simulink model "Squelette_DSPB_ModulateurOQPSK"  (R2016a)
settings: Solver=FixedStepDiscrete  StartTime=0.0  StopTime=1e-3  RelTol=1e-3
InitFcn:
  | %% DSPBuilder Start
  | alt_dspbuilder_update_model(bdroot)
  | %% DSPBuilder End
libraries: allblocks_alteradspbuilder2 x243
(part 1 of 2)
settings Model: Creator=rhev2401  LastModifiedBy=cous2509
settings DataIOCC: LimitDataPoints=on  SaveFormat=Array  SignalLoggingSaveFormat=ModelDataLogs
settings DebuggingCC: SolverPrmCheckMsg=warning  MultiTaskDSMMsg=warning  MultiTaskCondExecSysMsg=none
settings HardwareCC: ProdBitPerPointer=32  ProdLargestAtomicFloat=None  ProdIntDivRoundTo=Undefined  ProdEndianess=Unspecified  ProdWordSize=32  ProdHWDeviceType=32-bit Generic
settings ModelReferenceCC: PropagateSignalLabelsOutOfModel=off
settings ConfigComp: CovModelRefEnable=Off  CovSFcnEnable=off

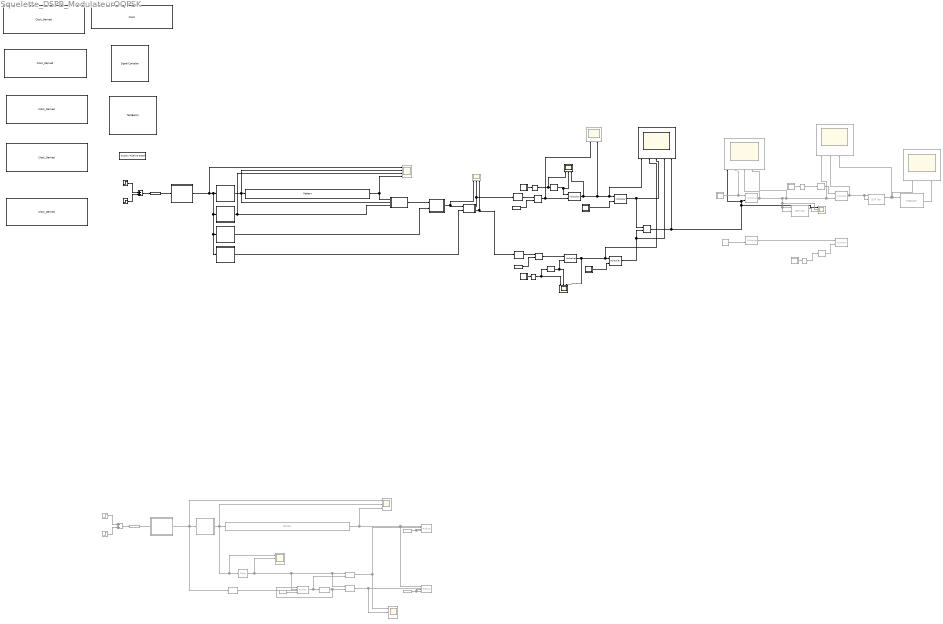
== system Squelette_DSPB_ModulateurOQPSK ==
  note: Transformation de la trame
  note: Rail Q O-QPSK
  note: Rail I O-QPSK
  note: Simulates an event to begin a transmission
  note: Bouton 01
  note: On se crée une impulsion qui dure la longueur de la trame.
      |
      | En vrai, il faudrait transmettre jusqu'à ce que le buffer soit vide...
  note: Paquet à transmettre (chips)
  note: Chipclock
  note: Notez que, pour ce programme, on a choisi d'utiliser la fréquence d'horloge de 100MHz.
  note: Si le dernier chip est rentré sur I, le prochain rentre sur Q, et vice-versa; génération de deux horloges d'1 MHz déphasées
  note: Cette boîte à délai compense pour le délai de la boîte "Pattern" (notez que la sortie de la boîte pattern commence 1 coup de clock après l'apparition du Enable)
  note: Si le dernier chip est rentré sur I, le prochain rentre sur Q, et vice-versa; génération de deux horloges d'1 MHz déphasées
  note: Simulates an event to begin a transmission
  note: 0000000000000000000000000000000011100101 10010000111011111111001101110100000101101110010100110001010100001010000110000110
      | 0 0 0 0 0 0 0 0 7 A 9 0 7 F F C E 2 8 6 7 A C 8 A 0 5 8 1 6
  note: Bouton 01
  note: On se crée une impulsion qui dure la longueur de la trame.
      |
      | En vrai, il faudrait transmettre jusqu'à ce que le buffer soit vide...
  note: Paquet à transmettre
  note: Bitclock
  note: Notez que, pour ce programme, on a choisi d'utiliser la fréquence d'horloge de 100MHz.
  note: Bit to symbol
  note: Symbol to chip
  note: Chip to I/Q
  1MHz Pulse Generator2 : Subsystem
  250kHz Pulse Generator : Subsystem
  2MHz Pulse Generator : Subsystem  Commented=on
  2MHz Pulse Generator2 : Subsystem
  62.5kHz Pulse Generator1 : Subsystem
  Add : Sum  Commented=on
  Add1 : Sum
  Bit to symbol : Subsystem
  Bouton : Subsystem  Commented=on
  Bouton1 : Subsystem
  Chip to I/Q : Subsystem
  Clock_100MHz : allblocks_alteradspbuilder2/Clock_Derived  ClockNumerator=1  ClockDenominator=2  ResetLatency=0  ResetRegisterCascadeDepth=0  SimulationStartCycle=5  PhaseOffset=0  Reset=aclr_100MHz  ResetType=Active Low  Export=off
  Clock_125MHz : allblocks_alteradspbuilder2/Clock_Derived  ClockNumerator=10  ClockDenominator=25  ResetLatency=0  ResetRegisterCascadeDepth=0  SimulationStartCycle=5  PhaseOffset=0  Reset=aclr_125MHz  ResetType=Active Low  Export=off
  Clock_1MHz : allblocks_alteradspbuilder2/Clock_Derived  ClockNumerator=50  ClockDenominator=1  ResetLatency=0  ResetRegisterCascadeDepth=0  SimulationStartCycle=5  PhaseOffset=0  Reset=aclr_1MHz  ResetType=Active Low  Export=off
  Clock_2MHz : allblocks_alteradspbuilder2/Clock_Derived  ClockNumerator=25  ClockDenominator=1  ResetLatency=0  ResetRegisterCascadeDepth=0  SimulationStartCycle=5  PhaseOffset=0  Reset=aclr_2MHz  ResetType=Active Low  Export=off
  Clock_50MHz : allblocks_alteradspbuilder2/Clock  ClockPeriod=20  ClockPeriodUnit=ns  SampleTime=20e-9  ResetLatency=0  ResetRegisterCascadeDepth=0  SimulationStartCycle=5  PhaseOffset=0  Reset=aclr  ResetType=Active Low  Export=off
  Clock_62p5MHz : allblocks_alteradspbuilder2/Clock_Derived  ClockNumerator=800  ClockDenominator=1  ResetLatency=0  ResetRegisterCascadeDepth=0  SimulationStartCycle=5  PhaseOffset=0  Reset=aclr_62p5MHz  ResetType=Active Low  Export=off
  Constant : allblocks_alteradspbuilder2/Constant  Commented=on  mask_cst=1  BusType=Signed Integer  bwl=8  bwr=0  roundMode=Truncate  satMode=Wrap  SpecifyClock=off  allowFloatingPointOverride=on  logOutputs=off  logFile=U:\S6\Projet\Squelette_ModulateurOQPSK__ORIG\tb_Squelette_DSPB_ModulateurOQPSK\Squelette%5FDSPB%5FModulateurOQPSK_Constant.fixedpointlog
  Constant1 : allblocks_alteradspbuilder2/Constant  Commented=on  mask_cst=1  BusType=Signed Integer  bwl=8  bwr=0  roundMode=Truncate  satMode=Wrap  SpecifyClock=off  allowFloatingPointOverride=on  logOutputs=off  logFile=U:\S6\Projet\Squelette_ModulateurOQPSK__ORIG\tb_Squelette_DSPB_ModulateurOQPSK\Squelette%5FDSPB%5FModulateurOQPSK_Constant1.fixedpointlog
  Constant2 : allblocks_alteradspbuilder2/Constant  Commented=on  mask_cst=1  BusType=Signed Integer  bwl=8  bwr=0  roundMode=Truncate  satMode=Wrap  SpecifyClock=off  allowFloatingPointOverride=on  logOutputs=off  logFile=U:\S6\Projet\Squelette_ModulateurOQPSK__ORIG\tb_Squelette_DSPB_ModulateurOQPSK\Squelette%5FDSPB%5FModulateurOQPSK_Constant2.fixedpointlog
  Constant3 : allblocks_alteradspbuilder2/Constant  mask_cst=-1  BusType=Signed Integer  bwl=8  bwr=4  roundMode=Truncate  satMode=Wrap  SpecifyClock=on  clock=Clock_100MHz  allowFloatingPointOverride=on  logOutputs=off  logFile=U:\S6\Projet\Squelette_ModulateurOQPSK__ORIG\tb_Squelette_DSPB_ModulateurOQPSK\Squelette%5FDSPB%5FModulateurOQPSK_Constant3.fixedpointlog
  Constant5 : allblocks_alteradspbuilder2/Constant  mask_cst=-1  BusType=Signed Integer  bwl=8  bwr=4  roundMode=Truncate  satMode=Wrap  SpecifyClock=on  clock=Clock_100MHz  allowFloatingPointOverride=on  logOutputs=off  logFile=U:\S6\Projet\Squelette_ModulateurOQPSK__ORIG\tb_Squelette_DSPB_ModulateurOQPSK\Squelette%5FDSPB%5FModulateurOQPSK_Constant5.fixedpointlog
  Coswave : Subsystem
  Coswave1 : Subsystem  Commented=on
  Delay : allblocks_alteradspbuilder2/Delay  Commented=on  pipeline=1  pipeline_display=1  ClockPhase=1  use_ena=off  use_sclr=off  allowFloatingPointOverride=on  logOutputs=off  logFile=U:\S6\Projet\Squelette_ModulateurOQPSK__ORIG\tb_Squelette_DSPB_ModulateurOQPSK\Squelette%5FDSPB%5FModulateurOQPSK_Delay.fixedpointlog  use_init=off  reset_value=1
  Delay1 : allblocks_alteradspbuilder2/Delay  pipeline=5  pipeline_display=5  ClockPhase=1  use_ena=off  use_sclr=off  allowFloatingPointOverride=on  logOutputs=off  logFile=U:\S6\Projet\Squelette_ModulateurOQPSK__ORIG\tb_Squelette_DSPB_ModulateurOQPSK\Squelette%5FDSPB%5FModulateurOQPSK_Delay1.fixedpointlog  use_init=off  reset_value=1
  Delay2 : allblocks_alteradspbuilder2/Delay  Commented=on  pipeline=5  pipeline_display=5  ClockPhase=1  use_ena=off  use_sclr=off  allowFloatingPointOverride=on  logOutputs=off  logFile=U:\S6\Projet\Squelette_ModulateurOQPSK__ORIG\tb_Squelette_DSPB_ModulateurOQPSK\Squelette%5FDSPB%5FModulateurOQPSK_Delay2.fixedpointlog  use_init=off  reset_value=1
  Delay3 : allblocks_alteradspbuilder2/Delay  Commented=on  pipeline=55  pipeline_display=55  ClockPhase=1  use_ena=off  use_sclr=off  allowFloatingPointOverride=on  logOutputs=off  logFile=U:\S6\Projet\Squelette_ModulateurOQPSK__ORIG\tb_Squelette_DSPB_ModulateurOQPSK\Squelette%5FDSPB%5FModulateurOQPSK_Delay3.fixedpointlog  use_init=off  reset_value=1
  Delay4 : allblocks_alteradspbuilder2/Delay  pipeline=55  pipeline_display=55  ClockPhase=1  use_ena=off  use_sclr=off  allowFloatingPointOverride=on  logOutputs=off  logFile=U:\S6\Projet\Squelette_ModulateurOQPSK__ORIG\tb_Squelette_DSPB_ModulateurOQPSK\Squelette%5FDSPB%5FModulateurOQPSK_Delay4.fixedpointlog  use_init=off  reset_value=1
  Display Pipeline Depth : allblocks_alteradspbuilder2/Display Pipeline Depth  DisplayLatencyOnBlocks=on
  Flipflop : allblocks_alteradspbuilder2/Flipflop  Commented=on  mode=DFFE  BusType=Single Bit  bwl=2  bwr=2  pipeline_display=1
  Flipflop1 : allblocks_alteradspbuilder2/Flipflop  Commented=on  mode=DFFE  BusType=Single Bit  bwl=2  bwr=2  pipeline_display=1
  Flipflop2 : allblocks_alteradspbuilder2/Flipflop  Commented=on  mode=DFFE  BusType=Single Bit  bwl=2  bwr=2  pipeline_display=1
  Gain : allblocks_alteradspbuilder2/Gain  vgain=2  BusType=Signed Integer  bwl=6  bwr=0  pipeline=0  pipeline_display=0  allowFloatingPointOverride=on  logOutputs=off  logFile=U:\S6\Projet\Squelette_ModulateurOQPSK__ORIG\tb_Squelette_DSPB_ModulateurOQPSK\Squelette%5FDSPB%5FModulateurOQPSK_Gain.fixedpointlog  use_ena=off  use_aclr=off  lpm=off  MaskValue=1
  Gain1 : allblocks_alteradspbuilder2/Gain  vgain=2  BusType=Signed Integer  bwl=6  bwr=0  pipeline=0  pipeline_display=0  allowFloatingPointOverride=on  logOutputs=off  logFile=U:\S6\Projet\Squelette_ModulateurOQPSK__ORIG\tb_Squelette_DSPB_ModulateurOQPSK\Squelette%5FDSPB%5FModulateurOQPSK_Gain1.fixedpointlog  use_ena=off  use_aclr=off  lpm=off  MaskValue=1
  Input : allblocks_alteradspbuilder2/Input  Commented=on  iofile=U:\S6\Projet\Squelette_ModulateurOQPSK__ORIG\tb_Squelette_DSPB_ModulateurOQPSK\Squelette%5FDSPB%5FModulateurOQPSK_Input.salt  BusType=Single Bit  bwl=1  bwr=0  SpecifyClock=on  clock=Clock_100MHz  PORTTYPE=Input  externalType=Inferred  allowFloatingPointOverride=on  logOutputs=off
  Input1 : allblocks_alteradspbuilder2/Input  iofile=U:\S6\Projet\Squelette_ModulateurOQPSK__ORIG\tb_Squelette_DSPB_ModulateurOQPSK\Squelette%5FDSPB%5FModulateurOQPSK_Input1.salt  BusType=Single Bit  bwl=1  bwr=0  SpecifyClock=on  clock=Clock_100MHz  PORTTYPE=Input  externalType=Inferred  allowFloatingPointOverride=on  logOutputs=off
  Integrator : allblocks_alteradspbuilder2/Integrator  Commented=on  bwl=32  depth=32  pipeline_display=32  use_ena=off  use_sclr=on  allowFloatingPointOverride=on  logOutputs=off  logFile=U:\S6\Projet\Squelette_ModulateurOQPSK__ORIG\tb_Squelette_DSPB_ModulateurOQPSK\Squelette%5FDSPB%5FModulateurOQPSK_Integrator.fixedpointlog
  Logical Bit Operator : allblocks_alteradspbuilder2/Logical Bit Operator  Commented=on  LogicalOperator=NOT  user_inputs=2  pipeline_display=0
  Logical Bit Operator1 : allblocks_alteradspbuilder2/Logical Bit Operator  Commented=on  LogicalOperator=AND  user_inputs=2  pipeline_display=0
  Logical Bit Operator2 : allblocks_alteradspbuilder2/Logical Bit Operator  Commented=on  LogicalOperator=AND  user_inputs=2  pipeline_display=0
  Logical Bit Operator3 : allblocks_alteradspbuilder2/Logical Bit Operator  Commented=on  LogicalOperator=NOT  user_inputs=2  pipeline_display=0
  Magnitude : allblocks_alteradspbuilder2/Magnitude  pipeline_display=0
  Magnitude1 : allblocks_alteradspbuilder2/Magnitude  pipeline_display=0
  Magnitude2 : allblocks_alteradspbuilder2/Magnitude  Commented=on  pipeline_display=0
  Magnitude3 : allblocks_alteradspbuilder2/Magnitude  Commented=on  pipeline_display=0
  Multiplier : allblocks_alteradspbuilder2/Multiplier  BusType=Signed Fractional  bwl=20  bwr=20  pipeline=0  pipeline_display=0  allowFloatingPointOverride=on  logOutputs=off  logFile=U:\S6\Projet\Squelette_ModulateurOQPSK__ORIG\tb_Squelette_DSPB_ModulateurOQPSK\Squelette%5FDSPB%5FModulateurOQPSK_Multiplier.fixedpointlog  UseEqualInputWidth=on  bbwl=8  bbwr=0  FullResolution=on  OutputMsb=8  OutputLsb=0  OutputBwl=16  OutputBwr=16  UseDedicatedCircuitry=YES  use_ena=off  use_aclr=off
  Multiplier1 : allblocks_alteradspbuilder2/Multiplier  BusType=Signed Fractional  bwl=20  bwr=20  pipeline=0  pipeline_display=0  allowFloatingPointOverride=on  logOutputs=off  logFile=U:\S6\Projet\Squelette_ModulateurOQPSK__ORIG\tb_Squelette_DSPB_ModulateurOQPSK\Squelette%5FDSPB%5FModulateurOQPSK_Multiplier1.fixedpointlog  UseEqualInputWidth=on  bbwl=8  bbwr=0  FullResolution=on  OutputMsb=8  OutputLsb=0  OutputBwl=16  OutputBwr=16  UseDedicatedCircuitry=YES  use_ena=off  use_aclr=off
  Multiplier2 : allblocks_alteradspbuilder2/Multiplier  BusType=Signed Fractional  bwl=20  bwr=20  pipeline=0  pipeline_display=0  allowFloatingPointOverride=on  logOutputs=off  logFile=U:\S6\Projet\Squelette_ModulateurOQPSK__ORIG\tb_Squelette_DSPB_ModulateurOQPSK\Squelette%5FDSPB%5FModulateurOQPSK_Multiplier2.fixedpointlog  UseEqualInputWidth=on  bbwl=8  bbwr=0  FullResolution=on  OutputMsb=8  OutputLsb=0  OutputBwl=16  OutputBwr=16  UseDedicatedCircuitry=YES  use_ena=off  use_aclr=off
  Multiplier3 : allblocks_alteradspbuilder2/Multiplier  BusType=Signed Fractional  bwl=20  bwr=20  pipeline=0  pipeline_display=0  allowFloatingPointOverride=on  logOutputs=off  logFile=U:\S6\Projet\Squelette_ModulateurOQPSK__ORIG\tb_Squelette_DSPB_ModulateurOQPSK\Squelette%5FDSPB%5FModulateurOQPSK_Multiplier3.fixedpointlog  UseEqualInputWidth=on  bbwl=8  bbwr=0  FullResolution=on  OutputMsb=8  OutputLsb=0  OutputBwl=16  OutputBwr=16  UseDedicatedCircuitry=YES  use_ena=off  use_aclr=off
  Multiplier4 : allblocks_alteradspbuilder2/Multiplier  Commented=on  BusType=Signed Fractional  bwl=20  bwr=20  pipeline=0  pipeline_display=0  allowFloatingPointOverride=on  logOutputs=off  logFile=U:\S6\Projet\Squelette_ModulateurOQPSK__ORIG\tb_Squelette_DSPB_ModulateurOQPSK\Squelette%5FDSPB%5FModulateurOQPSK_Multiplier4.fixedpointlog  UseEqualInputWidth=on  bbwl=8  bbwr=0  FullResolution=on  OutputMsb=8  OutputLsb=0  OutputBwl=16  OutputBwr=16  UseDedicatedCircuitry=YES  use_ena=off  use_aclr=off
  Multiplier5 : allblocks_alteradspbuilder2/Multiplier  Commented=on  BusType=Signed Fractional  bwl=20  bwr=20  pipeline=0  pipeline_display=0  allowFloatingPointOverride=on  logOutputs=off  logFile=U:\S6\Projet\Squelette_ModulateurOQPSK__ORIG\tb_Squelette_DSPB_ModulateurOQPSK\Squelette%5FDSPB%5FModulateurOQPSK_Multiplier5.fixedpointlog  UseEqualInputWidth=on  bbwl=8  bbwr=0  FullResolution=on  OutputMsb=8  OutputLsb=0  OutputBwl=16  OutputBwr=16  UseDedicatedCircuitry=YES  use_ena=off  use_aclr=off
  Multiplier6 : allblocks_alteradspbuilder2/Multiplier  Commented=on  BusType=Signed Fractional  bwl=20  bwr=20  pipeline=0  pipeline_display=0  allowFloatingPointOverride=on  logOutputs=off  logFile=U:\S6\Projet\Squelette_ModulateurOQPSK__ORIG\tb_Squelette_DSPB_ModulateurOQPSK\Squelette%5FDSPB%5FModulateurOQPSK_Multiplier6.fixedpointlog  UseEqualInputWidth=on  bbwl=8  bbwr=0  FullResolution=on  OutputMsb=8  OutputLsb=0  OutputBwl=16  OutputBwr=16  UseDedicatedCircuitry=YES  use_ena=off  use_aclr=off
  Multiplier7 : allblocks_alteradspbuilder2/Multiplier  Commented=on  BusType=Signed Fractional  bwl=20  bwr=20  pipeline=0  pipeline_display=0  allowFloatingPointOverride=on  logOutputs=off  logFile=U:\S6\Projet\Squelette_ModulateurOQPSK__ORIG\tb_Squelette_DSPB_ModulateurOQPSK\Squelette%5FDSPB%5FModulateurOQPSK_Multiplier7.fixedpointlog  UseEqualInputWidth=on  bbwl=8  bbwr=0  FullResolution=on  OutputMsb=8  OutputLsb=0  OutputBwl=16  OutputBwr=16  UseDedicatedCircuitry=YES  use_ena=off  use_aclr=off
  Parallel Adder Subtractor : allblocks_alteradspbuilder2/Parallel Adder Subtractor  number_of_inputs=2  direction=+  use_pipeline=off  pipeline_display=0  phase_selection=1  use_ena=off  use_aclr=off  allowFloatingPointOverride=on  logOutputs=off  logFile=U:\S6\Projet\Squelette_ModulateurOQPSK__ORIG\tb_Squelette_DSPB_ModulateurOQPSK\Squelette%5FDSPB%5FModulateurOQPSK_Parallel+Adder+Subtractor.fixedpointlog
  Parallel Adder Subtractor1 : allblocks_alteradspbuilder2/Parallel Adder Subtractor  number_of_inputs=2  direction=+  use_pipeline=off  pipeline_display=0  phase_selection=1  use_ena=off  use_aclr=off  allowFloatingPointOverride=on  logOutputs=off  logFile=U:\S6\Projet\Squelette_ModulateurOQPSK__ORIG\tb_Squelette_DSPB_ModulateurOQPSK\Squelette%5FDSPB%5FModulateurOQPSK_Parallel+Adder+Subtractor1.fixedpointlog
  Parallel Adder Subtractor2 : allblocks_alteradspbuilder2/Parallel Adder Subtractor  number_of_inputs=2  direction=+  use_pipeline=off  pipeline_display=0  phase_selection=1  use_ena=off  use_aclr=off  allowFloatingPointOverride=on  logOutputs=off  logFile=U:\S6\Projet\Squelette_ModulateurOQPSK__ORIG\tb_Squelette_DSPB_ModulateurOQPSK\Squelette%5FDSPB%5FModulateurOQPSK_Parallel+Adder+Subtractor2.fixedpointlog
  Pattern1 : allblocks_alteradspbuilder2/Pattern  Commented=on  Sequence=10011010111100001100110000110011  SpecifyClock=off  clock=Clock_250kHz  use_ena=on  use_sclr=off
  Pattern2 : allblocks_alteradspbuilder2/Pattern  Sequence=<binary blob, 120 chars, not shown>  SpecifyClock=off  clock=Clock_250kHz  use_ena=on  use_sclr=off
  SOP Tap : allblocks_alteradspbuilder2/SOP Tap  Commented=on  BusType=Unsigned Integer  bwl=8  bwr=0  number_of_taps=2  pipeline_display=2  use_ena=off  use_aclr=off  allowFloatingPointOverride=on  logOutputs=off  logFile=U:\S6\Projet\Squelette_ModulateurOQPSK__ORIG\tb_Squelette_DSPB_ModulateurOQPSK\Squelette%5FDSPB%5FModulateurOQPSK_SOP+Tap%3A%3Aq.fixedpointlog,U:\S6\Projet\Squelette_ModulateurOQPSK__ORIG\tb_Squelette_DSPB_ModulateurOQPSK\Squelette%5FDSPB%5FModulateurOQPSK_SOP+Tap%3A%3Adout.fixedpointlog,
  SOP Tap1 : allblocks_alteradspbuilder2/SOP Tap  Commented=on  BusType=Unsigned Integer  bwl=8  bwr=0  number_of_taps=2  pipeline_display=2  use_ena=off  use_aclr=off  allowFloatingPointOverride=on  logOutputs=off  logFile=U:\S6\Projet\Squelette_ModulateurOQPSK__ORIG\tb_Squelette_DSPB_ModulateurOQPSK\Squelette%5FDSPB%5FModulateurOQPSK_SOP+Tap1%3A%3Aq.fixedpointlog,U:\S6\Projet\Squelette_ModulateurOQPSK__ORIG\tb_Squelette_DSPB_ModulateurOQPSK\Squelette%5FDSPB%5FModulateurOQPSK_SOP+Tap1%3A%3Adout.fixedpointlog,
  Scope{,2,4,6} (4 alike) : Scope  Commented=on  NumInputPorts=3
  Scope1 : Scope  NumInputPorts=5
  Scope10 : Scope  Commented=on  NumInputPorts=5
  Scope11 : Scope  Commented=on  NumInputPorts=2
  Scope12 : Scope  Commented=on  NumInputPorts=4
  Scope3 : Scope  Commented=on  NumInputPorts=2
  Scope5 : Scope  Commented=on  NumInputPorts=4
  Scope7 : Scope  NumInputPorts=3
  Scope8 : Scope  NumInputPorts=3
  Scope9 : Scope  Commented=on  NumInputPorts=4
  Signal Compiler : allblocks_alteradspbuilder2/Signal Compiler  DeviceFamily=Cyclone V  DeviceName=AUTO  DisableEarlyHDLGeneration=off  EnableSignalTap=off  SignalTapDepth=128  UseBoardBlock=off  StpUseDefaultClock=on  StpClock=Clock_50MHz  ExportDir=C:\Users\pivd2501\Documents  MAX10_ProgrammingMode=Internal Flash (SDM) Single Boot
  Sinewave : Subsystem
  Sinewave1 : Subsystem
  Sinewave2 : Subsystem
  Sinewave3 : Subsystem  Commented=on
  Sinewave5 : Subsystem  Commented=on
  Sinewave6 : Subsystem  Commented=on
  Step : Step  Commented=on  Time=100e-6  Before=1  After=0  SampleTime=1/100e06  VectorParams1D=off
  Step1 : Step  Commented=on  Time=200e-6  SampleTime=1/100e06  VectorParams1D=off
  Step2 : Step  Time=100e-6  Before=1  After=0  SampleTime=1/100e06  VectorParams1D=off
  Step3 : Step  Time=200e-6  SampleTime=1/100e06  VectorParams1D=off
  Symbol to chip : Subsystem
  TestBench : allblocks_alteradspbuilder2/TestBench  enable=on  advancedMode=on  modelSimGui=on  maxDisplayErrors=1000  mismatchErrorLevel=Error  simdatafile=U:\S6\Projet\Squelette_ModulateurOQPSK__ORIG\tb_Squelette_DSPB_ModulateurOQPSK\Squelette_DSPB_ModulateurOQPSK.simdata.tcl
  wires:
  Add/1 -> Input/1
  Step1/1 -> Add/2
  Step/1 -> Add/1
  2MHz Pulse Generator/1(Pulse 2MHz) -> Scope4/1, Delay/1, Pattern1/1, Scope/2  "ENA"
  Pattern1/1 -> Flipflop2/1, Flipflop1/1, Scope/3  "Chips"
  Bouton/1(CLR 480u) -> Logical Bit Operator/1, 2MHz Pulse Generator/1(CLR), Scope/1  "SCLR"
  Input/1 -> Bouton/1(Button Press)
  Flipflop/1 -> Logical Bit Operator1/2, Logical Bit Operator3/1
  Logical Bit Operator3/1 -> Flipflop/1, Logical Bit Operator2/2
  Logical Bit Operator1/1 -> Scope2/1, Flipflop1/2  "ChipClock_I"
  Constant/1 -> Flipflop1/4, Flipflop1/3
  Constant1/1 -> Flipflop2/3, Flipflop2/4
  Logical Bit Operator2/1 -> Scope2/2, Flipflop2/2  "ChipClock_Q"
  Logical Bit Operator/1 -> Flipflop/3
  Constant2/1 -> Flipflop/4
  Gain/1 -> Parallel Adder Subtractor/1
  Constant5/1 -> Parallel Adder Subtractor/2
  Gain1/1 -> Parallel Adder Subtractor1/1
  Constant3/1 -> Parallel Adder Subtractor1/2
  Delay/1 -> Flipflop/2, Logical Bit Operator2/1, Logical Bit Operator1/1, Scope4/2
  Add1/1 -> Input1/1
  Step3/1 -> Add1/2
  Step2/1 -> Add1/1
  250kHz Pulse Generator/1(Pulse 250kHz) -> Scope5/2, Bit to symbol/2(Pulse_250kHz), Pattern2/1  "ENA"
  Bouton1/1(CLR 480u) -> 1MHz Pulse Generator2/1(CLR), 2MHz Pulse Generator2/1(CLR), 62.5kHz Pulse Generator1/1(CLR), 250kHz Pulse Generator/1(CLR), Scope5/1  "SCLR"
  Input1/1 -> Bouton1/1(Button Press)
  Pattern2/1 -> Scope5/4, Bit to symbol/1(Paquet)  "DATA"
  62.5kHz Pulse Generator1/1(Pulse 62.5kHz) -> Bit to symbol/3(Pulse_62.5kHz), Scope5/3
  Bit to symbol/1(symbole) -> Symbol to chip/1(Symbole)
  2MHz Pulse Generator2/1(Pulse 2MHz) -> Symbol to chip/2("Pulse_2MHz ")
  Symbol to chip/1(O_Chips) -> Scope6/1, Chip to I/Q/1(Data)
  1MHz Pulse Generator2/1(Pulse 1MHz) -> Chip to I/Q/2(Pulse_1MHz)
  Chip to I/Q/2(Q) -> Gain1/1, Scope6/3  "Chip_I"
  Chip to I/Q/1(I) -> Scope6/2, Gain/1  "Chip_Q"
  Multiplier/1 -> Scope1/3, Parallel Adder Subtractor2/1  "I modulé"
  Multiplier1/1 -> Scope1/4, Parallel Adder Subtractor2/2  "Q modulé"
  Parallel Adder Subtractor2/1 -> Scope1/5, Scope10/1, Multiplier4/2, Scope12/1  "I + Q"
  Multiplier2/1 -> Scope7/3, Scope3/2, Scope1/1, Multiplier/1  "I formé"
  Magnitude/1 -> Scope7/2, Multiplier2/1
  Parallel Adder Subtractor/1 -> Scope3/1, Multiplier2/2
  Coswave/1(Out1) -> Multiplier/2
  Sinewave/1(Out1) -> Multiplier1/2
  Sinewave1/1(Out1) -> Delay4/1
  Magnitude1/1 -> Scope8/2, Multiplier3/2
  Parallel Adder Subtractor1/1 -> Multiplier3/1
  Multiplier3/1 -> Scope1/2, Multiplier1/1, Scope8/3  "Q formé"
  Sinewave2/1(Out1) -> Delay1/1
  Delay1/1 -> Scope7/1, Magnitude/1
  Delay4/1 -> Scope8/1, Magnitude1/1
  Sinewave3/1(Out1) -> Multiplier5/2
  Coswave1/1(Out1) -> Scope10/2, Multiplier4/1
  Multiplier5/1 -> Multiplier7/1
  Sinewave5/1(Out1) -> Delay2/1
  Sinewave6/1(Out1) -> Delay3/1
  Delay3/1 -> Magnitude3/1
  Magnitude3/1 -> Multiplier7/2
  Magnitude2/1 -> Multiplier6/1
  Delay2/1 -> Magnitude2/1
  Multiplier4/1 -> Scope12/2, SOP Tap1/2, SOP Tap1/1, Scope10/4, Scope9/1, Multiplier6/2, Scope10/3
  Integrator/1 -> Scope11/2
  Multiplier6/1 -> SOP Tap/2, SOP Tap/1, Scope9/2
  SOP Tap/1 -> Scope9/3, Integrator/1, Scope11/1
  SOP Tap1/1 -> Scope12/3

== system Squelette_DSPB_ModulateurOQPSK/1MHz Pulse Generator2 ==
  CLR : Inport
  Comparator : allblocks_alteradspbuilder2/Comparator  direction=a == b  pipeline_display=0  allowFloatingPointOverride=on  logOutputs=off  logFile=U:\S6\Projet\Squelette_ModulateurOQPSK__ORIG\tb_Squelette_DSPB_ModulateurOQPSK\Squelette%5FDSPB%5FModulateurOQPSK_1MHz+Pulse+Generator2_Comparator.fixedpointlog
  Constant : allblocks_alteradspbuilder2/Constant  mask_cst=0  BusType=Unsigned Integer  bwl=1  bwr=0  roundMode=Truncate  satMode=Wrap  SpecifyClock=off  allowFloatingPointOverride=on  logOutputs=off  logFile=U:\S6\Projet\Squelette_ModulateurOQPSK__ORIG\tb_Squelette_DSPB_ModulateurOQPSK\Squelette%5FDSPB%5FModulateurOQPSK_1MHz+Pulse+Generator2_Constant.fixedpointlog
  Constant1 : allblocks_alteradspbuilder2/Constant  mask_cst=1  BusType=Unsigned Integer  bwl=1  bwr=0  roundMode=Truncate  satMode=Wrap  SpecifyClock=off  allowFloatingPointOverride=on  logOutputs=off  logFile=U:\S6\Projet\Squelette_ModulateurOQPSK__ORIG\tb_Squelette_DSPB_ModulateurOQPSK\Squelette%5FDSPB%5FModulateurOQPSK_1MHz+Pulse+Generator2_Constant1.fixedpointlog
  Counter : allblocks_alteradspbuilder2/Counter  BusType=Unsigned Integer  bwl=10  bwr=0  use_modulo=on  modulo=100  SpecifyClock=off  direction=Increment  use_sload=off  use_sset=off  svalue=1  use_clk_ena=off  use_ena=off  use_sclr=on  pipeline_display=1
  Flipflop : allblocks_alteradspbuilder2/Flipflop  mode=DFFE  BusType=Single Bit  bwl=2  bwr=2  pipeline_display=1
  Logical Bit Operator1 : allblocks_alteradspbuilder2/Logical Bit Operator  LogicalOperator=AND  user_inputs=2  pipeline_display=0
  Logical Bit Operator2 : allblocks_alteradspbuilder2/Logical Bit Operator  LogicalOperator=NOT  user_inputs=2  pipeline_display=0
  Scope : Scope  Commented=on  NumInputPorts=2
  Scope1 : Scope  NumInputPorts=2
  Pulse 1MHz : Outport
  wires:
  Logical Bit Operator1/1 -> Flipflop/1, Scope1/1
  Constant1/1 -> Flipflop/2, Flipflop/3, Flipflop/4
  Flipflop/1 -> Pulse 1MHz/1, Scope1/2
  Comparator/1 -> Logical Bit Operator1/1
  Logical Bit Operator2/1 -> Logical Bit Operator1/2
  CLR/1 -> Counter/1, Scope/1, Logical Bit Operator2/1
  Constant/1 -> Comparator/2
  Counter/1 -> Comparator/1, Scope/2

== system Squelette_DSPB_ModulateurOQPSK/250kHz Pulse Generator ==
  CLR : Inport
  Comparator : allblocks_alteradspbuilder2/Comparator  direction=a == b  pipeline_display=0  allowFloatingPointOverride=on  logOutputs=off  logFile=U:\S6\Projet\Squelette_ModulateurOQPSK__ORIG\tb_Squelette_DSPB_ModulateurOQPSK\Squelette%5FDSPB%5FModulateurOQPSK_250kHz+Pulse+Generator_Comparator.fixedpointlog
  Constant : allblocks_alteradspbuilder2/Constant  mask_cst=0  BusType=Unsigned Integer  bwl=1  bwr=0  roundMode=Truncate  satMode=Wrap  SpecifyClock=off  allowFloatingPointOverride=on  logOutputs=off  logFile=U:\S6\Projet\Squelette_ModulateurOQPSK__ORIG\tb_Squelette_DSPB_ModulateurOQPSK\Squelette%5FDSPB%5FModulateurOQPSK_250kHz+Pulse+Generator_Constant.fixedpointlog
  Constant1 : allblocks_alteradspbuilder2/Constant  mask_cst=1  BusType=Unsigned Integer  bwl=1  bwr=0  roundMode=Truncate  satMode=Wrap  SpecifyClock=off  allowFloatingPointOverride=on  logOutputs=off  logFile=U:\S6\Projet\Squelette_ModulateurOQPSK__ORIG\tb_Squelette_DSPB_ModulateurOQPSK\Squelette%5FDSPB%5FModulateurOQPSK_250kHz+Pulse+Generator_Constant1.fixedpointlog
  Counter : allblocks_alteradspbuilder2/Counter  BusType=Unsigned Integer  bwl=10  bwr=0  use_modulo=on  modulo=400  SpecifyClock=off  direction=Increment  use_sload=off  use_sset=off  svalue=1  use_clk_ena=off  use_ena=off  use_sclr=on  pipeline_display=1
  Flipflop : allblocks_alteradspbuilder2/Flipflop  mode=DFFE  BusType=Single Bit  bwl=2  bwr=2  pipeline_display=1
  Logical Bit Operator1 : allblocks_alteradspbuilder2/Logical Bit Operator  LogicalOperator=AND  user_inputs=2  pipeline_display=0
  Logical Bit Operator2 : allblocks_alteradspbuilder2/Logical Bit Operator  LogicalOperator=NOT  user_inputs=2  pipeline_display=0
  Scope : Scope  Commented=on  NumInputPorts=2
  Pulse 250kHz : Outport
  wires:
  Counter/1 -> Scope/2, Comparator/1
  Constant/1 -> Comparator/2
  CLR/1 -> Logical Bit Operator2/1, Scope/1, Counter/1
  Logical Bit Operator2/1 -> Logical Bit Operator1/2
  Comparator/1 -> Logical Bit Operator1/1
  Flipflop/1 -> Pulse 250kHz/1
  Logical Bit Operator1/1 -> Flipflop/1
  Constant1/1 -> Flipflop/4, Flipflop/3, Flipflop/2

== system Squelette_DSPB_ModulateurOQPSK/2MHz Pulse Generator ==
  CLR : Inport
  Comparator : allblocks_alteradspbuilder2/Comparator  direction=a == b  pipeline_display=0  allowFloatingPointOverride=on  logOutputs=off  logFile=U:\ProjetS6\Squelette_ModulateurOQPSK__ORIG\tb_Squelette_DSPB_ModulateurOQPSK\Squelette%5FDSPB%5FModulateurOQPSK_2MHz+Pulse+Generator_Comparator.fixedpointlog
  Constant : allblocks_alteradspbuilder2/Constant  mask_cst=0  BusType=Unsigned Integer  bwl=1  bwr=0  roundMode=Truncate  satMode=Wrap  SpecifyClock=off  allowFloatingPointOverride=on  logOutputs=off  logFile=U:\ProjetS6\Squelette_ModulateurOQPSK__ORIG\tb_Squelette_DSPB_ModulateurOQPSK\Squelette%5FDSPB%5FModulateurOQPSK_2MHz+Pulse+Generator_Constant.fixedpointlog
  Constant1 : allblocks_alteradspbuilder2/Constant  mask_cst=1  BusType=Unsigned Integer  bwl=1  bwr=0  roundMode=Truncate  satMode=Wrap  SpecifyClock=off  allowFloatingPointOverride=on  logOutputs=off  logFile=U:\ProjetS6\Squelette_ModulateurOQPSK__ORIG\tb_Squelette_DSPB_ModulateurOQPSK\Squelette%5FDSPB%5FModulateurOQPSK_2MHz+Pulse+Generator_Constant1.fixedpointlog
  Counter : allblocks_alteradspbuilder2/Counter  BusType=Unsigned Integer  bwl=10  bwr=0  use_modulo=on  modulo=50  SpecifyClock=off  direction=Increment  use_sload=off  use_sset=off  svalue=1  use_clk_ena=off  use_ena=off  use_sclr=on  pipeline_display=1
  Flipflop : allblocks_alteradspbuilder2/Flipflop  mode=DFFE  BusType=Single Bit  bwl=2  bwr=2  pipeline_display=1
  Logical Bit Operator1 : allblocks_alteradspbuilder2/Logical Bit Operator  LogicalOperator=AND  user_inputs=2  pipeline_display=0
  Logical Bit Operator2 : allblocks_alteradspbuilder2/Logical Bit Operator  LogicalOperator=NOT  user_inputs=2  pipeline_display=0
  Scope : Scope  NumInputPorts=5
  Pulse 2MHz : Outport
  wires:
  Counter/1 -> Scope/1, Comparator/1
  Constant/1 -> Comparator/2
  CLR/1 -> Logical Bit Operator2/1, Scope/2, Counter/1
  Logical Bit Operator2/1 -> Logical Bit Operator1/2
  Comparator/1 -> Logical Bit Operator1/1
  Flipflop/1 -> Pulse 2MHz/1
  Logical Bit Operator1/1 -> Flipflop/1
  Constant1/1 -> Flipflop/4, Flipflop/3, Flipflop/2

== system Squelette_DSPB_ModulateurOQPSK/2MHz Pulse Generator2 ==
  CLR : Inport
  Comparator : allblocks_alteradspbuilder2/Comparator  direction=a == b  pipeline_display=0  allowFloatingPointOverride=on  logOutputs=off  logFile=U:\S6\Projet\Squelette_ModulateurOQPSK__ORIG\tb_Squelette_DSPB_ModulateurOQPSK\Squelette%5FDSPB%5FModulateurOQPSK_2MHz+Pulse+Generator2_Comparator.fixedpointlog
  Constant : allblocks_alteradspbuilder2/Constant  mask_cst=0  BusType=Unsigned Integer  bwl=1  bwr=0  roundMode=Truncate  satMode=Wrap  SpecifyClock=off  allowFloatingPointOverride=on  logOutputs=off  logFile=U:\S6\Projet\Squelette_ModulateurOQPSK__ORIG\tb_Squelette_DSPB_ModulateurOQPSK\Squelette%5FDSPB%5FModulateurOQPSK_2MHz+Pulse+Generator2_Constant.fixedpointlog
  Constant1 : allblocks_alteradspbuilder2/Constant  mask_cst=1  BusType=Unsigned Integer  bwl=1  bwr=0  roundMode=Truncate  satMode=Wrap  SpecifyClock=off  allowFloatingPointOverride=on  logOutputs=off  logFile=U:\S6\Projet\Squelette_ModulateurOQPSK__ORIG\tb_Squelette_DSPB_ModulateurOQPSK\Squelette%5FDSPB%5FModulateurOQPSK_2MHz+Pulse+Generator2_Constant1.fixedpointlog
  Counter : allblocks_alteradspbuilder2/Counter  BusType=Unsigned Integer  bwl=8  bwr=0  use_modulo=on  modulo=50  SpecifyClock=off  direction=Increment  use_sload=off  use_sset=off  svalue=1  use_clk_ena=off  use_ena=off  use_sclr=on  pipeline_display=1
  Flipflop : allblocks_alteradspbuilder2/Flipflop  mode=DFFE  BusType=Single Bit  bwl=2  bwr=2  pipeline_display=1
  Logical Bit Operator1 : allblocks_alteradspbuilder2/Logical Bit Operator  LogicalOperator=AND  user_inputs=2  pipeline_display=0
  Logical Bit Operator2 : allblocks_alteradspbuilder2/Logical Bit Operator  LogicalOperator=NOT  user_inputs=2  pipeline_display=0
  Scope : Scope  Commented=on  NumInputPorts=2
  Scope1 : Scope  NumInputPorts=2
  Pulse 2MHz : Outport
  wires:
  Counter/1 -> Scope/2, Comparator/1
  Constant/1 -> Comparator/2
  CLR/1 -> Logical Bit Operator2/1, Scope/1, Counter/1
  Logical Bit Operator2/1 -> Logical Bit Operator1/2
  Comparator/1 -> Logical Bit Operator1/1
  Flipflop/1 -> Scope1/2, Pulse 2MHz/1
  Constant1/1 -> Flipflop/4, Flipflop/3, Flipflop/2
  Logical Bit Operator1/1 -> Scope1/1, Flipflop/1

== system Squelette_DSPB_ModulateurOQPSK/62.5kHz Pulse Generator1 ==
  CLR : Inport
  Comparator : allblocks_alteradspbuilder2/Comparator  direction=a == b  pipeline_display=0  allowFloatingPointOverride=on  logOutputs=off  logFile=U:\S6\Projet\Squelette_ModulateurOQPSK__ORIG\tb_Squelette_DSPB_ModulateurOQPSK\Squelette%5FDSPB%5FModulateurOQPSK_62.5kHz+Pulse+Generator1_Comparator.fixedpointlog
  Constant : allblocks_alteradspbuilder2/Constant  mask_cst=0  BusType=Unsigned Integer  bwl=1  bwr=0  roundMode=Truncate  satMode=Wrap  SpecifyClock=off  allowFloatingPointOverride=on  logOutputs=off  logFile=U:\S6\Projet\Squelette_ModulateurOQPSK__ORIG\tb_Squelette_DSPB_ModulateurOQPSK\Squelette%5FDSPB%5FModulateurOQPSK_62.5kHz+Pulse+Generator1_Constant.fixedpointlog
  Constant1 : allblocks_alteradspbuilder2/Constant  mask_cst=1  BusType=Unsigned Integer  bwl=1  bwr=0  roundMode=Truncate  satMode=Wrap  SpecifyClock=off  allowFloatingPointOverride=on  logOutputs=off  logFile=U:\S6\Projet\Squelette_ModulateurOQPSK__ORIG\tb_Squelette_DSPB_ModulateurOQPSK\Squelette%5FDSPB%5FModulateurOQPSK_62.5kHz+Pulse+Generator1_Constant1.fixedpointlog
  Counter : allblocks_alteradspbuilder2/Counter  BusType=Unsigned Integer  bwl=12  bwr=0  use_modulo=on  modulo=1600  SpecifyClock=off  direction=Increment  use_sload=off  use_sset=off  svalue=1  use_clk_ena=off  use_ena=off  use_sclr=on  pipeline_display=1
  Flipflop : allblocks_alteradspbuilder2/Flipflop  mode=DFFE  BusType=Single Bit  bwl=2  bwr=2  pipeline_display=1
  Logical Bit Operator1 : allblocks_alteradspbuilder2/Logical Bit Operator  LogicalOperator=AND  user_inputs=2  pipeline_display=0
  Logical Bit Operator2 : allblocks_alteradspbuilder2/Logical Bit Operator  LogicalOperator=NOT  user_inputs=2  pipeline_display=0
  Scope : Scope  Commented=on  NumInputPorts=2
  Scope1 : Scope  NumInputPorts=2
  Pulse 62.5kHz : Outport
  wires:
  Counter/1 -> Scope/2, Comparator/1
  Constant/1 -> Comparator/2
  CLR/1 -> Logical Bit Operator2/1, Scope/1, Counter/1
  Logical Bit Operator2/1 -> Logical Bit Operator1/2
  Comparator/1 -> Logical Bit Operator1/1
  Flipflop/1 -> Scope1/2, Pulse 62.5kHz/1
  Constant1/1 -> Flipflop/4, Flipflop/3, Flipflop/2
  Logical Bit Operator1/1 -> Scope1/1, Flipflop/1

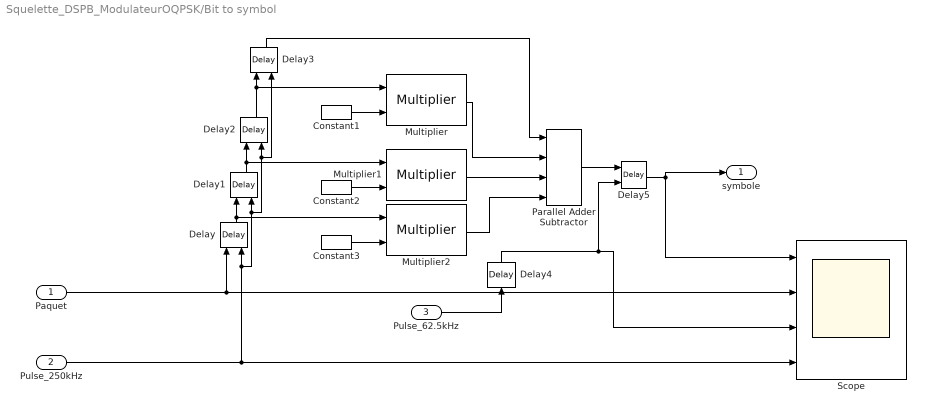
== system Squelette_DSPB_ModulateurOQPSK/Bit to symbol ==
  Paquet : Inport
  Pulse_250kHz : Inport  Port=2
  Pulse_62.5kHz : Inport  Port=3
  Constant1 : allblocks_alteradspbuilder2/Constant  mask_cst=2  BusType=Unsigned Integer  bwl=4  bwr=0  roundMode=Truncate  satMode=Wrap  SpecifyClock=off  allowFloatingPointOverride=on  logOutputs=off  logFile=U:\S6\Projet\Squelette_ModulateurOQPSK__ORIG\tb_Squelette_DSPB_ModulateurOQPSK\Squelette%5FDSPB%5FModulateurOQPSK_Bit+to+symbol_Constant1.fixedpointlog
  Constant2 : allblocks_alteradspbuilder2/Constant  mask_cst=4  BusType=Unsigned Integer  bwl=4  bwr=0  roundMode=Truncate  satMode=Wrap  SpecifyClock=off  allowFloatingPointOverride=on  logOutputs=off  logFile=U:\S6\Projet\Squelette_ModulateurOQPSK__ORIG\tb_Squelette_DSPB_ModulateurOQPSK\Squelette%5FDSPB%5FModulateurOQPSK_Bit+to+symbol_Constant2.fixedpointlog
  Constant3 : allblocks_alteradspbuilder2/Constant  mask_cst=8  BusType=Unsigned Integer  bwl=4  bwr=0  roundMode=Truncate  satMode=Wrap  SpecifyClock=off  allowFloatingPointOverride=on  logOutputs=off  logFile=U:\S6\Projet\Squelette_ModulateurOQPSK__ORIG\tb_Squelette_DSPB_ModulateurOQPSK\Squelette%5FDSPB%5FModulateurOQPSK_Bit+to+symbol_Constant3.fixedpointlog
  Delay : allblocks_alteradspbuilder2/Delay  pipeline=1  pipeline_display=1  ClockPhase=1  use_ena=on  use_sclr=off  allowFloatingPointOverride=on  logOutputs=off  logFile=U:\S6\Projet\Squelette_ModulateurOQPSK__ORIG\tb_Squelette_DSPB_ModulateurOQPSK\Squelette%5FDSPB%5FModulateurOQPSK_Bit+to+symbol_Delay.fixedpointlog  use_init=off  reset_value=1
  Delay1 : allblocks_alteradspbuilder2/Delay  pipeline=1  pipeline_display=1  ClockPhase=1  use_ena=on  use_sclr=off  allowFloatingPointOverride=on  logOutputs=off  logFile=U:\S6\Projet\Squelette_ModulateurOQPSK__ORIG\tb_Squelette_DSPB_ModulateurOQPSK\Squelette%5FDSPB%5FModulateurOQPSK_Bit+to+symbol_Delay1.fixedpointlog  use_init=off  reset_value=1
  Delay2 : allblocks_alteradspbuilder2/Delay  pipeline=1  pipeline_display=1  ClockPhase=1  use_ena=on  use_sclr=off  allowFloatingPointOverride=on  logOutputs=off  logFile=U:\S6\Projet\Squelette_ModulateurOQPSK__ORIG\tb_Squelette_DSPB_ModulateurOQPSK\Squelette%5FDSPB%5FModulateurOQPSK_Bit+to+symbol_Delay2.fixedpointlog  use_init=off  reset_value=1
  Delay3 : allblocks_alteradspbuilder2/Delay  pipeline=1  pipeline_display=1  ClockPhase=1  use_ena=on  use_sclr=off  allowFloatingPointOverride=on  logOutputs=off  logFile=U:\S6\Projet\Squelette_ModulateurOQPSK__ORIG\tb_Squelette_DSPB_ModulateurOQPSK\Squelette%5FDSPB%5FModulateurOQPSK_Bit+to+symbol_Delay3.fixedpointlog  use_init=off  reset_value=1
  Delay4 : allblocks_alteradspbuilder2/Delay  pipeline=1  pipeline_display=1  ClockPhase=1  use_ena=off  use_sclr=off  allowFloatingPointOverride=on  logOutputs=off  logFile=U:\S6\Projet\Squelette_ModulateurOQPSK__ORIG\tb_Squelette_DSPB_ModulateurOQPSK\Squelette%5FDSPB%5FModulateurOQPSK_Bit+to+symbol_Delay4.fixedpointlog  use_init=off  reset_value=1
  Delay5 : allblocks_alteradspbuilder2/Delay  pipeline=1  pipeline_display=1  ClockPhase=1  use_ena=on  use_sclr=off  allowFloatingPointOverride=on  logOutputs=off  logFile=U:\S6\Projet\Squelette_ModulateurOQPSK__ORIG\tb_Squelette_DSPB_ModulateurOQPSK\Squelette%5FDSPB%5FModulateurOQPSK_Bit+to+symbol_Delay5.fixedpointlog  use_init=off  reset_value=1
  Multiplier : allblocks_alteradspbuilder2/Multiplier  BusType=Unsigned Integer  bwl=1  bwr=0  pipeline=0  pipeline_display=0  allowFloatingPointOverride=on  logOutputs=off  logFile=U:\S6\Projet\Squelette_ModulateurOQPSK__ORIG\tb_Squelette_DSPB_ModulateurOQPSK\Squelette%5FDSPB%5FModulateurOQPSK_Bit+to+symbol_Multiplier.fixedpointlog  UseEqualInputWidth=off  bbwl=2  bbwr=0  FullResolution=on  OutputMsb=8  OutputLsb=0  OutputBwl=16  OutputBwr=16  UseDedicatedCircuitry=YES  use_ena=off  use_aclr=off
  Multiplier1 : allblocks_alteradspbuilder2/Multiplier  BusType=Unsigned Integer  bwl=1  bwr=0  pipeline=0  pipeline_display=0  allowFloatingPointOverride=on  logOutputs=off  logFile=U:\S6\Projet\Squelette_ModulateurOQPSK__ORIG\tb_Squelette_DSPB_ModulateurOQPSK\Squelette%5FDSPB%5FModulateurOQPSK_Bit+to+symbol_Multiplier1.fixedpointlog  UseEqualInputWidth=off  bbwl=3  bbwr=0  FullResolution=on  OutputMsb=8  OutputLsb=0  OutputBwl=16  OutputBwr=16  UseDedicatedCircuitry=YES  use_ena=off  use_aclr=off
  Multiplier2 : allblocks_alteradspbuilder2/Multiplier  BusType=Unsigned Integer  bwl=1  bwr=0  pipeline=0  pipeline_display=0  allowFloatingPointOverride=on  logOutputs=off  logFile=U:\S6\Projet\Squelette_ModulateurOQPSK__ORIG\tb_Squelette_DSPB_ModulateurOQPSK\Squelette%5FDSPB%5FModulateurOQPSK_Bit+to+symbol_Multiplier2.fixedpointlog  UseEqualInputWidth=off  bbwl=4  bbwr=0  FullResolution=on  OutputMsb=8  OutputLsb=0  OutputBwl=16  OutputBwr=16  UseDedicatedCircuitry=YES  use_ena=off  use_aclr=off
  Parallel Adder Subtractor : allblocks_alteradspbuilder2/Parallel Adder Subtractor  number_of_inputs=4  direction=+  use_pipeline=off  pipeline_display=0  phase_selection=1  use_ena=on  use_aclr=off  allowFloatingPointOverride=on  logOutputs=off  logFile=U:\S6\Projet\Squelette_ModulateurOQPSK__ORIG\tb_Squelette_DSPB_ModulateurOQPSK\Squelette%5FDSPB%5FModulateurOQPSK_Bit+to+symbol_Parallel+Adder+Subtractor.fixedpointlog
  Scope : Scope  NumInputPorts=4
  symbole : Outport
  wires:
  Pulse_250kHz/1 -> Delay3/2, Delay2/2, Delay1/2, Delay/2, Scope/4
  Paquet/1 -> Delay/1, Scope/2
  Delay2/1 -> Multiplier/1, Delay3/1
  Constant1/1 -> Multiplier/2
  Delay1/1 -> Multiplier1/1, Delay2/1
  Constant2/1 -> Multiplier1/2
  Delay/1 -> Delay1/1, Multiplier2/1
  Constant3/1 -> Multiplier2/2
  Pulse_62.5kHz/1 -> Delay4/1
  Delay5/1 -> Scope/1, symbole/1
  Multiplier/1 -> Parallel Adder Subtractor/2
  Multiplier1/1 -> Parallel Adder Subtractor/3
  Multiplier2/1 -> Parallel Adder Subtractor/4
  Delay4/1 -> Scope/3, Delay5/2
  Parallel Adder Subtractor/1 -> Delay5/1
  Delay3/1 -> Parallel Adder Subtractor/1

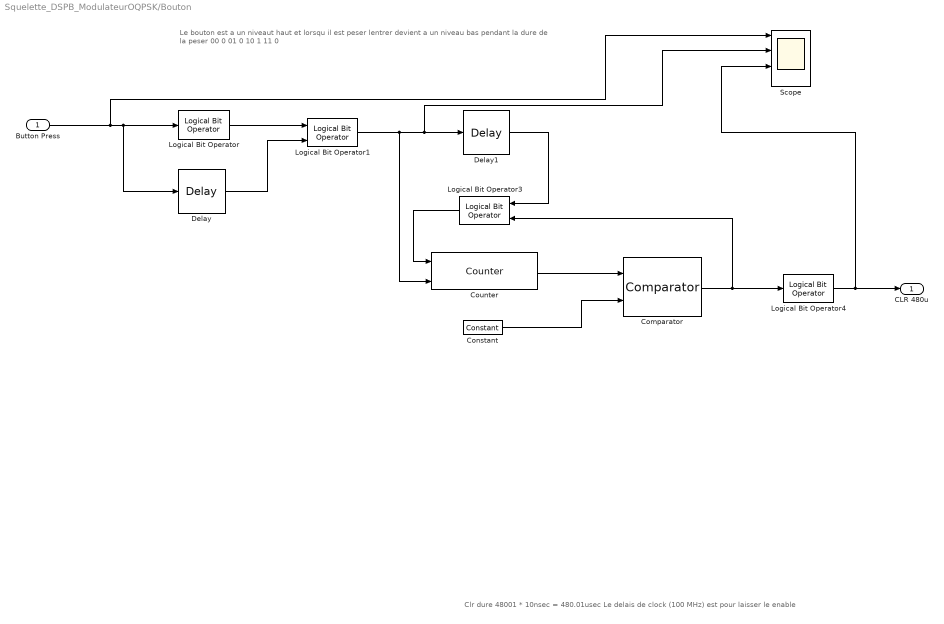
== system Squelette_DSPB_ModulateurOQPSK/Bouton ==
  note: Clr dure 48001 * 10nsec = 480.01usec Le delais de clock (100 MHz) est pour laisser le enable
  note: Le bouton est a un niveaut haut et lorsqu il est peser lentrer devient a un niveau bas pendant la dure de la peser
      |
      | 00  0
      | 01  0
      | 10  1
      | 11  0
  Button Press : Inport
  Comparator : allblocks_alteradspbuilder2/Comparator  direction=a >= b  pipeline_display=0  allowFloatingPointOverride=on  logOutputs=off  logFile=U:\ProjetS6\Squelette_ModulateurOQPSK__ORIG\tb_Squelette_DSPB_ModulateurOQPSK\Squelette%5FDSPB%5FModulateurOQPSK_Bouton_Comparator.fixedpointlog
  Constant : allblocks_alteradspbuilder2/Constant  mask_cst=1  BusType=Unsigned Integer  bwl=8  bwr=0  roundMode=Truncate  satMode=Wrap  SpecifyClock=off  allowFloatingPointOverride=on  logOutputs=off  logFile=U:\ProjetS6\Squelette_ModulateurOQPSK__ORIG\tb_Squelette_DSPB_ModulateurOQPSK\Squelette%5FDSPB%5FModulateurOQPSK_Bouton_Constant.fixedpointlog
  Counter : allblocks_alteradspbuilder2/Counter  BusType=Unsigned Integer  bwl=16  bwr=0  use_modulo=on  modulo=48001  SpecifyClock=off  clock=Clock_100MHz  direction=Increment  use_sload=off  use_sset=off  svalue=1  use_clk_ena=off  use_ena=on  use_sclr=on  pipeline_display=1
  Delay : allblocks_alteradspbuilder2/Delay  pipeline=1  pipeline_display=1  ClockPhase=1  use_ena=off  use_sclr=off  allowFloatingPointOverride=on  logOutputs=off  logFile=U:\ProjetS6\Squelette_ModulateurOQPSK__ORIG\tb_Squelette_DSPB_ModulateurOQPSK\Squelette%5FDSPB%5FModulateurOQPSK_Bouton_Delay.fixedpointlog  use_init=off  reset_value=1
  Delay1 : allblocks_alteradspbuilder2/Delay  pipeline=1  pipeline_display=1  ClockPhase=1  use_ena=off  use_sclr=off  allowFloatingPointOverride=on  logOutputs=off  logFile=U:\ProjetS6\Squelette_ModulateurOQPSK__ORIG\tb_Squelette_DSPB_ModulateurOQPSK\Squelette%5FDSPB%5FModulateurOQPSK_Bouton_Delay1.fixedpointlog  use_init=off  reset_value=1
  Logical Bit Operator : allblocks_alteradspbuilder2/Logical Bit Operator  LogicalOperator=NOT  user_inputs=2  pipeline_display=0
  Logical Bit Operator1 : allblocks_alteradspbuilder2/Logical Bit Operator  LogicalOperator=AND  user_inputs=2  pipeline_display=0
  Logical Bit Operator3 : allblocks_alteradspbuilder2/Logical Bit Operator  LogicalOperator=OR  user_inputs=2  pipeline_display=0
  Logical Bit Operator4 : allblocks_alteradspbuilder2/Logical Bit Operator  LogicalOperator=NOT  user_inputs=2  pipeline_display=0
  Scope : Scope  NumInputPorts=4
  CLR 480u : Outport
  wires:
  Button Press/1 -> Scope/1, Logical Bit Operator/1, Delay/1
  Logical Bit Operator/1 -> Logical Bit Operator1/1
  Logical Bit Operator1/1 -> Scope/2, Delay1/1, Counter/2
  Counter/1 -> Comparator/1
  Constant/1 -> Comparator/2
  Delay1/1 -> Logical Bit Operator3/1
  Logical Bit Operator3/1 -> Counter/1
  Comparator/1 -> Logical Bit Operator3/2, Logical Bit Operator4/1
  Delay/1 -> Logical Bit Operator1/2
  Logical Bit Operator4/1 -> Scope/3, CLR 480u/1

== system Squelette_DSPB_ModulateurOQPSK/Bouton1 ==
  note: Clr dure 48001 * 10nsec = 480.01usec Le delais de clock (100 MHz) est pour laisser le enable
  note: Le bouton est a un niveaut haut et lorsqu il est peser lentrer devient a un niveau bas pendant la dure de la peser
      |
      | 00  0
      | 01  0
      | 10  1
      | 11  0
  Button Press : Inport
  Comparator : allblocks_alteradspbuilder2/Comparator  direction=a >= b  pipeline_display=0  allowFloatingPointOverride=on  logOutputs=off  logFile=U:\S6\Projet\Squelette_ModulateurOQPSK__ORIG\tb_Squelette_DSPB_ModulateurOQPSK\Squelette%5FDSPB%5FModulateurOQPSK_Bouton1_Comparator.fixedpointlog
  Constant : allblocks_alteradspbuilder2/Constant  mask_cst=1  BusType=Unsigned Integer  bwl=8  bwr=0  roundMode=Truncate  satMode=Wrap  SpecifyClock=off  allowFloatingPointOverride=on  logOutputs=off  logFile=U:\S6\Projet\Squelette_ModulateurOQPSK__ORIG\tb_Squelette_DSPB_ModulateurOQPSK\Squelette%5FDSPB%5FModulateurOQPSK_Bouton1_Constant.fixedpointlog
  Counter : allblocks_alteradspbuilder2/Counter  BusType=Unsigned Integer  bwl=16  bwr=0  use_modulo=on  modulo=48001  SpecifyClock=off  clock=Clock_100MHz  direction=Increment  use_sload=off  use_sset=off  svalue=1  use_clk_ena=off  use_ena=on  use_sclr=on  pipeline_display=1
  Delay : allblocks_alteradspbuilder2/Delay  pipeline=1  pipeline_display=1  ClockPhase=1  use_ena=off  use_sclr=off  allowFloatingPointOverride=on  logOutputs=off  logFile=U:\S6\Projet\Squelette_ModulateurOQPSK__ORIG\tb_Squelette_DSPB_ModulateurOQPSK\Squelette%5FDSPB%5FModulateurOQPSK_Bouton1_Delay.fixedpointlog  use_init=off  reset_value=1
  Delay1 : allblocks_alteradspbuilder2/Delay  pipeline=1  pipeline_display=1  ClockPhase=1  use_ena=off  use_sclr=off  allowFloatingPointOverride=on  logOutputs=off  logFile=U:\S6\Projet\Squelette_ModulateurOQPSK__ORIG\tb_Squelette_DSPB_ModulateurOQPSK\Squelette%5FDSPB%5FModulateurOQPSK_Bouton1_Delay1.fixedpointlog  use_init=off  reset_value=1
  Logical Bit Operator : allblocks_alteradspbuilder2/Logical Bit Operator  LogicalOperator=NOT  user_inputs=2  pipeline_display=0
  Logical Bit Operator1 : allblocks_alteradspbuilder2/Logical Bit Operator  LogicalOperator=AND  user_inputs=2  pipeline_display=0
  Logical Bit Operator3 : allblocks_alteradspbuilder2/Logical Bit Operator  LogicalOperator=OR  user_inputs=2  pipeline_display=0
  Logical Bit Operator4 : allblocks_alteradspbuilder2/Logical Bit Operator  LogicalOperator=NOT  user_inputs=2  pipeline_display=0
  Scope : Scope  Commented=on  NumInputPorts=3
  CLR 480u : Outport
  wires:
  Button Press/1 -> Scope/1, Logical Bit Operator/1, Delay/1
  Logical Bit Operator/1 -> Logical Bit Operator1/1
  Logical Bit Operator1/1 -> Scope/2, Delay1/1, Counter/2
  Counter/1 -> Comparator/1
  Constant/1 -> Comparator/2
  Delay1/1 -> Logical Bit Operator3/1
  Logical Bit Operator3/1 -> Counter/1
  Comparator/1 -> Logical Bit Operator3/2, Logical Bit Operator4/1
  Delay/1 -> Logical Bit Operator1/2
  Logical Bit Operator4/1 -> Scope/3, CLR 480u/1

== system Squelette_DSPB_ModulateurOQPSK/Chip to I//Q ==
  Data : Inport
  Pulse_1MHz : Inport  Port=2
  Constant1 : allblocks_alteradspbuilder2/Constant  mask_cst=1  BusType=Unsigned Integer  bwl=1  bwr=0  roundMode=Truncate  satMode=Wrap  SpecifyClock=off  allowFloatingPointOverride=on  logOutputs=off  logFile=U:\S6\Projet\Squelette_ModulateurOQPSK__ORIG\tb_Squelette_DSPB_ModulateurOQPSK\Squelette%5FDSPB%5FModulateurOQPSK_Chip+to+I__Q_Constant1.fixedpointlog
  Constant3 : allblocks_alteradspbuilder2/Constant  mask_cst=1  BusType=Unsigned Integer  bwl=1  bwr=0  roundMode=Truncate  satMode=Wrap  SpecifyClock=off  allowFloatingPointOverride=on  logOutputs=off  logFile=U:\S6\Projet\Squelette_ModulateurOQPSK__ORIG\tb_Squelette_DSPB_ModulateurOQPSK\Squelette%5FDSPB%5FModulateurOQPSK_Chip+to+I__Q_Constant3.fixedpointlog
  Delay : allblocks_alteradspbuilder2/Delay  pipeline=51  pipeline_display=51  ClockPhase=1  use_ena=off  use_sclr=off  allowFloatingPointOverride=on  logOutputs=off  logFile=U:\S6\Projet\Squelette_ModulateurOQPSK__ORIG\tb_Squelette_DSPB_ModulateurOQPSK\Squelette%5FDSPB%5FModulateurOQPSK_Chip+to+I__Q_Delay.fixedpointlog  use_init=off  reset_value=1
  Delay1 : allblocks_alteradspbuilder2/Delay  pipeline=1  pipeline_display=1  ClockPhase=1  use_ena=off  use_sclr=off  allowFloatingPointOverride=on  logOutputs=off  logFile=U:\S6\Projet\Squelette_ModulateurOQPSK__ORIG\tb_Squelette_DSPB_ModulateurOQPSK\Squelette%5FDSPB%5FModulateurOQPSK_Chip+to+I__Q_Delay1.fixedpointlog  use_init=off  reset_value=1
  Flipflop : allblocks_alteradspbuilder2/Flipflop  mode=DFFE  BusType=Single Bit  bwl=2  bwr=2  pipeline_display=1
  Flipflop1 : allblocks_alteradspbuilder2/Flipflop  mode=DFFE  BusType=Single Bit  bwl=2  bwr=2  pipeline_display=1
  Scope6 : Scope  NumInputPorts=3
  I : Outport
  Q : Outport  Port=2
  wires:
  Constant3/1 -> Flipflop1/4, Flipflop1/3
  Constant1/1 -> Flipflop/4, Flipflop/3
  Flipflop/1 -> I/1
  Data/1 -> Flipflop1/1, Scope6/1, Flipflop/1
  Delay/1 -> Scope6/3, Flipflop1/2
  Flipflop1/1 -> Q/1
  Pulse_1MHz/1 -> Delay/1, Delay1/1
  Delay1/1 -> Scope6/2, Flipflop/2
